simulink model "Practica1_pendulo"  (R2025a)
settings: Solver=ode45  StartTime=0.0  StopTime=10  RelTol=1e-3
undefined symbols (not defined in the file): adot0, alpha0, Beq, Bp, Fc, g, Ip, lp, Mc, Mp, x0, xdot0

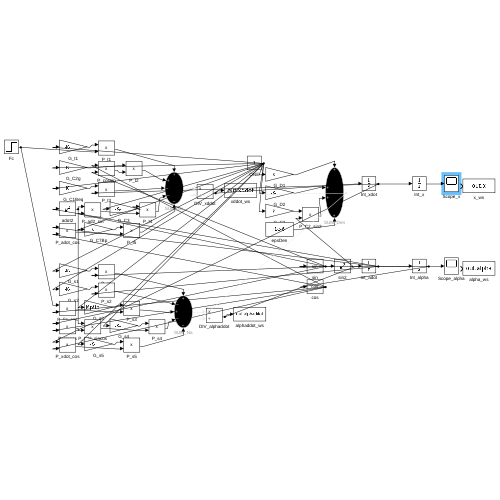
[thumbnail: Simulink's stored preview of the top-level diagram]
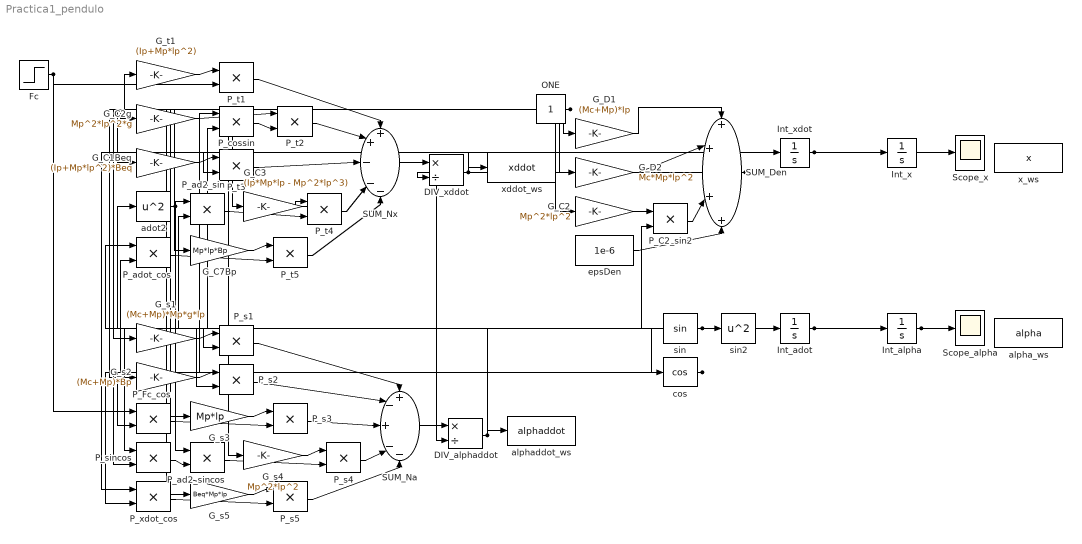
== system Practica1_pendulo ==
  DIV_alphaddot : Product  Inputs=*/
  DIV_xddot : Product  Inputs=*/
  Fc : Step  Time=0  After=Fc  SampleTime=0
  G_C1Beq : Gain  Gain=(Ip+Mp*lp^2)*Beq
  G_C2 : Gain  Gain=Mp^2*lp^2
  G_C2g : Gain  Gain=Mp^2*lp^2*g
  G_C3 : Gain  Gain=(Ip*Mp*lp - Mp^2*lp^3)
  G_C7Bp : Gain  Gain=Mp*lp*Bp
  G_D1 : Gain  Gain=(Mc+Mp)*Ip
  G_D2 : Gain  Gain=Mc*Mp*lp^2
  G_s1 : Gain  Gain=(Mc+Mp)*Mp*g*lp
  G_s2 : Gain  Gain=(Mc+Mp)*Bp
  G_s3 : Gain  Gain=Mp*lp
  G_s4 : Gain  Gain=Mp^2*lp^2
  G_s5 : Gain  Gain=Beq*Mp*lp
  G_t1 : Gain  Gain=(Ip+Mp*lp^2)
  Int_adot : Integrator  InitialCondition=adot0
  Int_alpha : Integrator  InitialCondition=alpha0
  Int_x : Integrator  InitialCondition=x0
  Int_xdot : Integrator  InitialCondition=xdot0
  ONE : Constant
  P_C2_sin2 : Product
  P_Fc_cos : Product
  P_ad2_sin : Product
  P_ad2_sincos : Product
  P_adot_cos : Product
  P_cossin : Product
  P_s{1..5} (5 alike) : Product
  P_sincos : Product
  P_t{1..5} (5 alike) : Product
  P_xdot_cos : Product
  SUM_Den : Sum  Inputs=++++
  SUM_Na : Sum  Inputs=+-+--
  SUM_Nx : Sum  Inputs=++---
  Scope_alpha : Scope
      settings: ActiveDisplayYMinimum=-3.7453039697730617  ActiveDisplayYMaximum=33.882268653157
  Scope_x : Scope
      settings: ActiveDisplayYMinimum=-0.019331422269881934  ActiveDisplayYMaximum=0.17398280042893743
  adot2 : Math  Operator=square
  alpha_ws : ToWorkspace  VariableName=alpha  SampleTime=-1
  alphaddot_ws : ToWorkspace  VariableName=alphaddot  SampleTime=-1
  cos : Trigonometry  Operator=cos
  epsDen : Constant  Value=1e-6
  sin : Trigonometry
  sin2 : Math  Operator=square
  x_ws : ToWorkspace  VariableName=x  SampleTime=-1
  xddot_ws : ToWorkspace  VariableName=xddot  SampleTime=-1
  wires:
  Int_x/1 -> Scope_x/1
  Int_alpha/1 -> Scope_alpha/1, sin/1, cos/1
  sin/1 -> sin2/1, P_cossin/2, P_ad2_sin/2, P_s1/2, P_sincos/1
  ONE/1 -> G_D1/1, G_D2/1, G_C2/1, G_t1/1, G_C2g/1, G_C1Beq/1, G_C3/1, G_C7Bp/1, G_s1/1, G_s2/1, G_s3/1, G_s4/1, G_s5/1
  G_C2/1 -> P_C2_sin2/1
  sin2/1 -> P_C2_sin2/2
  G_D1/1 -> SUM_Den/1
  G_D2/1 -> SUM_Den/2
  P_C2_sin2/1 -> SUM_Den/3
  epsDen/1 -> SUM_Den/4
  G_t1/1 -> P_t1/1
  Fc/1 -> P_t1/2, P_Fc_cos/1
  cos/1 -> P_cossin/1, P_adot_cos/2, P_Fc_cos/2, P_sincos/2, P_xdot_cos/2
  G_C2g/1 -> P_t2/1
  P_cossin/1 -> P_t2/2
  G_C1Beq/1 -> P_t3/1
  Int_xdot/1 -> P_t3/2, Int_x/1, P_xdot_cos/1
  Int_adot/1 -> adot2/1, P_adot_cos/1, P_s2/2, Int_alpha/1
  adot2/1 -> P_ad2_sin/1, P_ad2_sincos/1
  G_C3/1 -> P_t4/1
  P_ad2_sin/1 -> P_t4/2
  G_C7Bp/1 -> P_t5/1
  P_adot_cos/1 -> P_t5/2
  P_t1/1 -> SUM_Nx/1
  P_t2/1 -> SUM_Nx/2
  P_t3/1 -> SUM_Nx/3
  P_t4/1 -> SUM_Nx/4
  P_t5/1 -> SUM_Nx/5
  SUM_Nx/1 -> DIV_xddot/1
  SUM_Den/1 -> DIV_xddot/2, DIV_alphaddot/2
  DIV_xddot/1 -> Int_xdot/1, xddot_ws/1
  G_s1/1 -> P_s1/1
  G_s2/1 -> P_s2/1
  G_s3/1 -> P_s3/1
  P_Fc_cos/1 -> P_s3/2
  P_sincos/1 -> P_ad2_sincos/2
  G_s4/1 -> P_s4/1
  P_ad2_sincos/1 -> P_s4/2
  G_s5/1 -> P_s5/1
  P_xdot_cos/1 -> P_s5/2
  P_s1/1 -> SUM_Na/1
  P_s2/1 -> SUM_Na/2
  P_s3/1 -> SUM_Na/3
  P_s4/1 -> SUM_Na/4
  P_s5/1 -> SUM_Na/5
  SUM_Na/1 -> DIV_alphaddot/1
  DIV_alphaddot/1 -> Int_adot/1, alphaddot_ws/1
